simulink model "multiplier_test"  (R2018b)
settings: Solver=VariableStepAuto  StartTime=0.0  StopTime=10.0  RelTol=1e-3
settings Model: Creator=annat  LastModifiedBy=annat

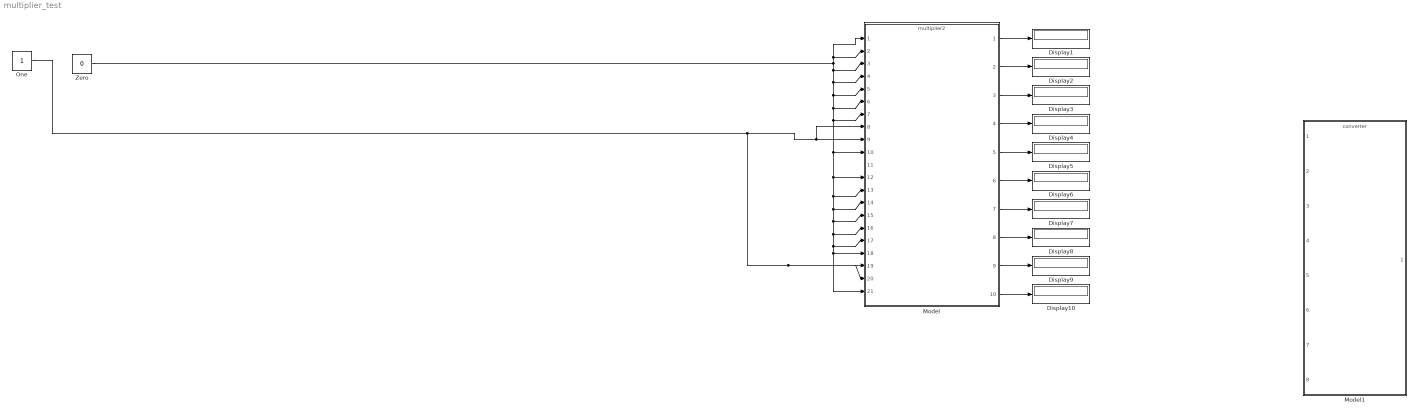
== system multiplier_test ==
  Display{1..10} (10 alike) : Display
      settings: Decimation=5
  Model : ModelReference  ModelNameDialog=multiplier2  SimulationMode=Normal  ModelReferenceVersion=1.12
  Model1 : ModelReference  ModelNameDialog=converter  SimulationMode=Normal  ModelReferenceVersion=1.7
  One : Constant  OutDataTypeStr=Inherit: Inherit via back propagation
  Zero : Constant  Value=0  OutDataTypeStr=Inherit: Inherit via back propagation
  wires:
  Zero/1 -> Model/1, Model/2, Model/5, Model/12, Model/15, Model/16, Model/17, Model/21, Model/18, Model/14, Model/13, Model/10, Model/7, Model/6, Model/4, Model/3
  Model/1 -> Display1/1
  Model/2 -> Display2/1
  Model/3 -> Display3/1
  Model/4 -> Display4/1
  Model/5 -> Display5/1
  Model/6 -> Display6/1
  Model/7 -> Display7/1
  Model/8 -> Display8/1
  Model/9 -> Display9/1
  Model/10 -> Display10/1
  One/1 -> Model/19, Model/20, Model/8, Model/9
